simulink model "Final_Simulation"  (R2017a)
settings: Solver=FixedStepAuto  StartTime=0.0  StopTime=5  FixedStep=0.001  RelTol=1e-3
values from neighbouring files (symbols this model uses):
  dX0 = [30; 20]*(pi/180)    [CAD_data.m]
  Theta = Theta_Initial    [CAD_data.m]
  X0 = [90;50]*(pi/180)    [CAD_data.m]    (also in Reduced_Regressor_Verification.m)
settings Model: Creator=Hero  LastModifiedBy=Hero

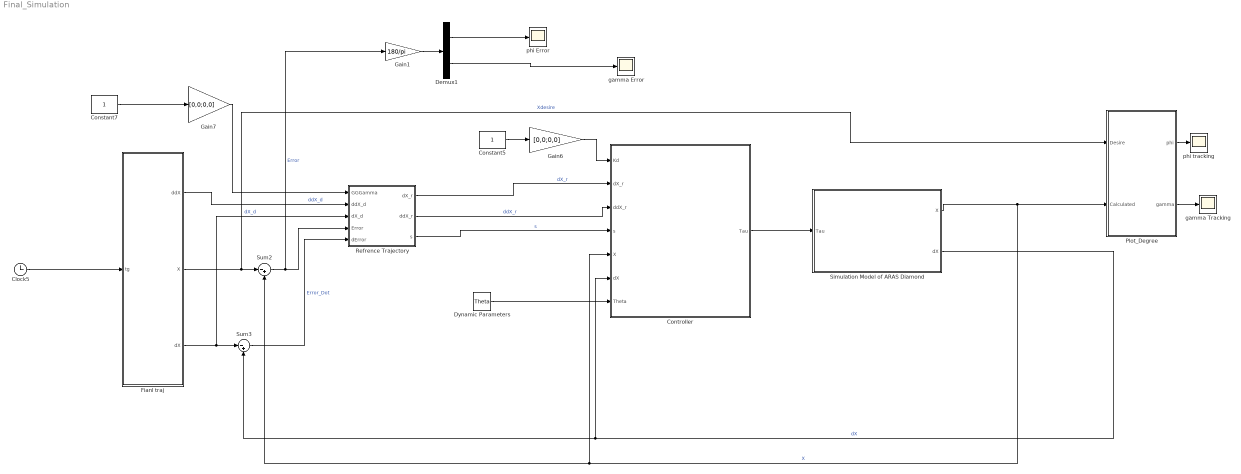
== system Final_Simulation ==
  Clock5 : Clock
  Constant5 : Constant
  Constant7 : Constant
  Controller : MATLAB Function  TreatAsAtomicUnit=on
  Demux1 : Demux  Outputs=2
  Dynamic Parameters : Constant  Value=Theta
  Fianl traj : MATLAB Function  TreatAsAtomicUnit=on
  Gain1 : Gain  Gain=180/pi
  Gain6 : Gain  Gain=[0,0;0,0]
  Gain7 : Gain  Gain=[0,0;0,0]
  Plot_Degree : Subsystem
  Refrence Trajectory : MATLAB Function  TreatAsAtomicUnit=on
  Simulation Model of ARAS Diamond : Subsystem
  Sum2 : Sum  Inputs=|-+
  Sum3 : Sum  Inputs=|-+
  gamma Error : Scope
  gamma Tracking : Scope
  phi Error : Scope
  phi tracking : Scope
  wires:
  Refrence Trajectory/2(ddX_r) -> Controller/3(ddX_r)  "ddX_r"
  Simulation Model of ARAS Diamond/1(X) -> Sum2/2, Controller/5(X), Plot_Degree/2(Calculated)  "X"
  Sum2/1 -> Gain1/1, Refrence Trajectory/4(Error)  "Error"
  Gain7/1 -> Refrence Trajectory/1(GGGamma)
  Fianl traj/1(ddX) -> Refrence Trajectory/2(ddX_d)  "ddX_d"
  Clock5/1 -> Fianl traj/1(tg)
  Constant5/1 -> Gain6/1
  Constant7/1 -> Gain7/1
  Refrence Trajectory/1(dX_r) -> Controller/2(dX_r)  "dX_r"
  Gain6/1 -> Controller/1(Kd)
  Refrence Trajectory/3(s) -> Controller/4(s)  "s"
  Sum3/1 -> Refrence Trajectory/5(dError)  "Error_Dot"
  Fianl traj/3(dX) -> Refrence Trajectory/3(dX_d), Sum3/1  "dX_d"
  Simulation Model of ARAS Diamond/2(dX) -> Sum3/2, Controller/6(dX)  "dX"
  Fianl traj/2(X) -> Sum2/1, Plot_Degree/1(Desire)  "Xdesire"
  Plot_Degree/2(gamma) -> gamma Tracking/1
  Plot_Degree/1(phi) -> phi tracking/1
  Demux1/2 -> gamma Error/1
  Demux1/1 -> phi Error/1
  Controller/1(Tau) -> Simulation Model of ARAS Diamond/1(Tau)
  Gain1/1 -> Demux1/1
  Dynamic Parameters/1 -> Controller/7(Theta)

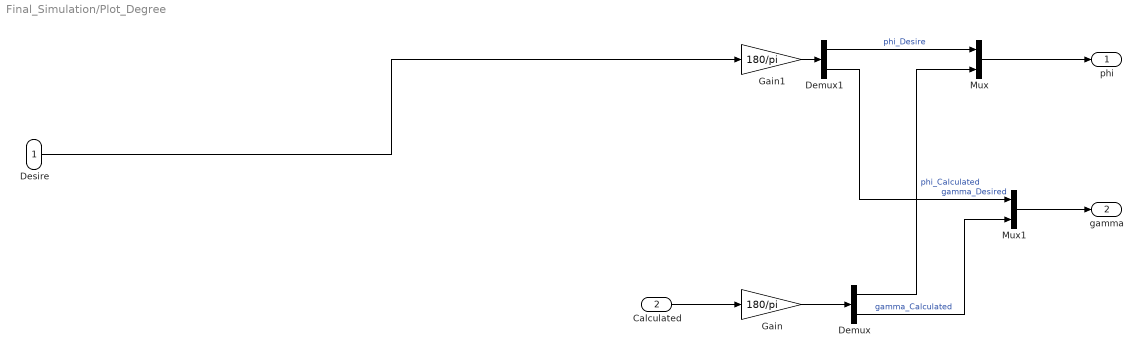
== system Final_Simulation/Plot_Degree ==
  Desire : Inport
  Calculated : Inport  Port=2
  Demux : Demux  Outputs=2
  Demux1 : Demux  Outputs=2
  Gain : Gain  Gain=180/pi
  Gain1 : Gain  Gain=180/pi
  Mux : Mux  Inputs=2
  Mux1 : Mux  Inputs=2
  phi : Outport
  gamma : Outport  Port=2
  wires:
  Mux/1 -> phi/1
  Demux/1 -> Mux/2  "phi_Calculated"
  Gain1/1 -> Demux1/1
  Mux1/1 -> gamma/1
  Demux1/1 -> Mux/1  "phi_Desire"
  Demux1/2 -> Mux1/1  "gamma_Desired"
  Demux/2 -> Mux1/2  "gamma_Calculated"
  Desire/1 -> Gain1/1
  Calculated/1 -> Gain/1
  Gain/1 -> Demux/1

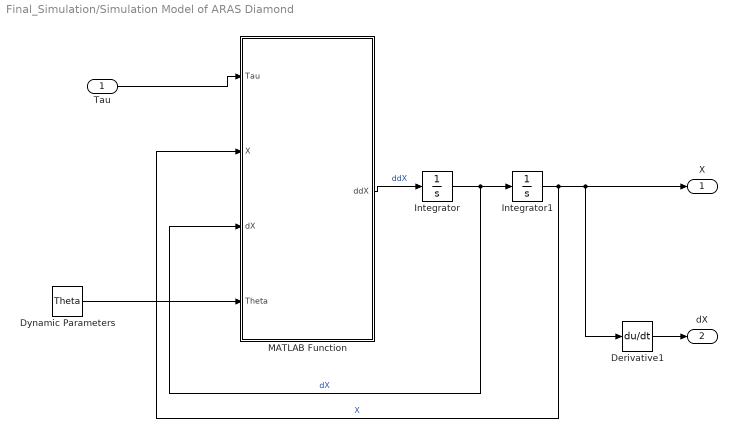
== system Final_Simulation/Simulation Model of ARAS Diamond ==
  Tau : Inport
  Derivative1 : Derivative
  Dynamic Parameters : Constant  Value=Theta
  Integrator : Integrator  InitialCondition=dX0
  Integrator1 : Integrator  InitialCondition=X0
  MATLAB Function : MATLAB Function  TreatAsAtomicUnit=on
  X : Outport
  dX : Outport  Port=2
  wires:
  Tau/1 -> MATLAB Function/1(Tau)
  MATLAB Function/1(ddX) -> Integrator/1  "ddX"
  Integrator/1 -> Integrator1/1, MATLAB Function/3(dX)  "dX"
  Integrator1/1 -> Derivative1/1, X/1, MATLAB Function/2(X)  "X"
  Derivative1/1 -> dX/1
  Dynamic Parameters/1 -> MATLAB Function/4(Theta)

== matlab function Final_Simulation/Controller ==
  data: Kd input; Tau output; dX_r input; ddX_r input; s input; X input; dX input; Theta input
function Tau  = fcn(Kd,dX_r,ddX_r,s,X,dX,Theta)


%% Adaptation Import
Theta1=Theta(1:9,1);Theta2=Theta(10:18,1);Theta3=Theta(19:27,1);Theta4=Theta(28:end,1);
Ibar1=Theta1(4:end,1);Ibar2=Theta2(4:end,1);Ibar3=Theta3(4:end,1);Ibar4=Theta4(4:end,1);
mrho1=Theta1(1:3,1);mrho2=Theta2(1:3,1);mrho3=Theta3(1:3,1);mrho4=Theta4(1:3,1);

% Model Import
M=Mass_Matrix_Adaptive(X,Ibar1,Ibar2,Ibar3,Ibar4);
C=C_Matrix_Adaptive(X,dX,Ibar1,Ibar2,Ibar3,Ibar4);
g=G_Matrix_Adaptive(X,mrho1,mrho2,mrho3,mrho4);


% M=Mass_Matrix(X);
% C=C_Matrix(X,dX);
% g=G_Matrix(X);
%% Control Law
F=M*ddX_r+C*dX_r+g-Kd*s;
J=Jacobian_Final(X);
Tau=J'\F;

%% >>>>>Reza for Verification 
% Ym=Slotine_Regressor(X,dX,dX_r,ddX_r);
% Error_Dy=(M*ddX_r+C*dX_r+g)-Ym*Theta;

end

== matlab function Final_Simulation/Refrence Trajectory ==
  data: GGGamma input; ddX_d input; dX_r output; dX_d input; Error input; dError input; ddX_r output; s output
function [dX_r,ddX_r,s] = fcn(GGGamma,ddX_d,dX_d,Error,dError)


dX_r=dX_d-GGGamma*Error;
ddX_r=ddX_d-GGGamma*dError;
s=dError+GGGamma*Error;

end

== matlab function Final_Simulation/Simulation Model of ARAS Diamond/MATLAB Function ==
  data: Tau input; ddX output; X input; dX input; Theta input
function ddX = fcn(Tau,X,dX,Theta)

%% Model Import
J=Jacobian_Final(X);
F=J'*Tau;

%% Adaptation Import
Theta1=Theta(1:9,1);Theta2=Theta(10:18,1);Theta3=Theta(19:27,1);Theta4=Theta(28:end,1);
Ibar1=Theta1(4:end,1);Ibar2=Theta2(4:end,1);Ibar3=Theta3(4:end,1);Ibar4=Theta4(4:end,1);
mrho1=Theta1(1:3,1);mrho2=Theta2(1:3,1);mrho3=Theta3(1:3,1);mrho4=Theta4(1:3,1);

% Model Import
M=Mass_Matrix_Adaptive(X,Ibar1,Ibar2,Ibar3,Ibar4);
C=C_Matrix_Adaptive(X,dX,Ibar1,Ibar2,Ibar3,Ibar4);
g=G_Matrix_Adaptive(X,mrho1,mrho2,mrho3,mrho4);


% M=Mass_Matrix(X);
% C=C_Matrix(X,dX);
% g=G_Matrix(X);

%% Forward Dynamics
ddX=(M^-1)*(F-C*dX-g);

end

== matlab function Final_Simulation/Fianl traj ==
  settings: updateMethod=DISCRETE
  data: ddX output; X output; dX output; tg input
function [ddX,X,dX]   = fcn(tg)

t=tg;

%% Trajectory Define (Sinusoidal)
X0=[90;50]*(pi/180);
X1=30*sin(t);X2=20*sin(t);
X=[X1;X2]*(pi/180)+X0;

dX1=30*cos(t);dX2=20*cos(t);
dX=[dX1;dX2]*(pi/180);

ddX1=-30*sin(t);ddX2=-20*sin(t);
ddX=[ddX1;ddX2]*(pi/180);

end
